simulink model "lqr_delay"  (R2017a)
settings: Solver=VariableStepAuto  StartTime=0.0  StopTime=4  RelTol=1e-3
values from neighbouring files (symbols this model uses):
  A_lq = [A7d B7d; 0 0 0 0]    [q13.m]
  B_lq = [0; 0; 0; 1]    [q13.m]
  C_lq = [C7d 0]    [q13.m]
  DCgain7 = D7d + C7cl*inv(eye(3)-A7cl)*B7d    [q13.m]    (also in q5.m; q5_reduced.m)
  DCgain_lq = D7d + C_lq_cl*inv(eye(4)-A_lq_cl)*B_lq    [q13.m]
  h7 = 0.08    [q13.m]    (also in q5.m = 0.006; q5_reduced.m)
undefined symbols (not defined in the file or in its folder): A7d, B7d, C7d, D5d, K7, K_lq
settings Model: Creator=Aleksandra  LastModifiedBy=Aleksandra

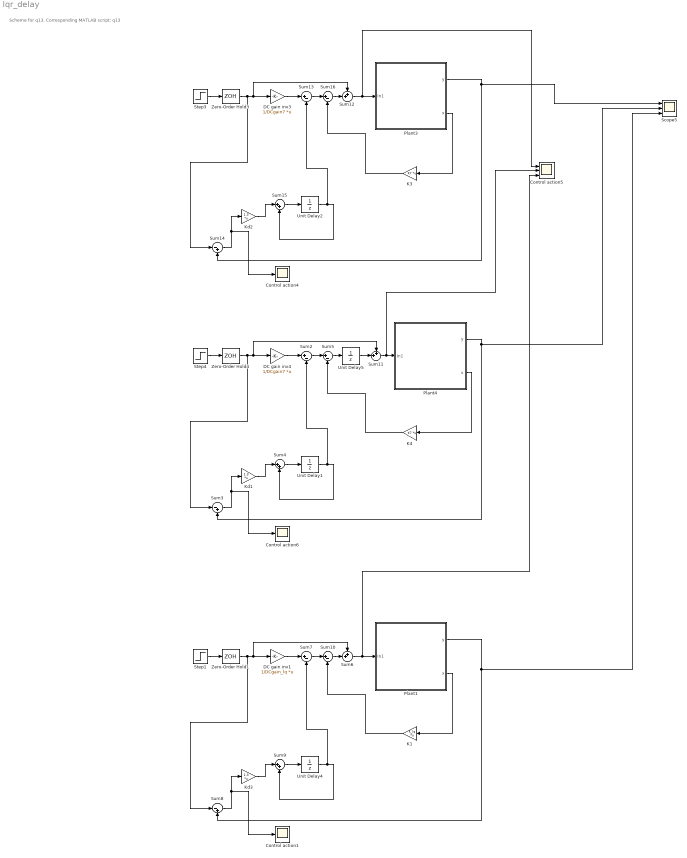
== system lqr_delay ==
  note: Scheme for q13.
      | Corresponding MATLAB script: q13
  Control action1 : Scope
  Control action4 : Scope
  Control action5 : Scope  NumInputPorts=3
  Control action6 : Scope
  DC gain inv1 : Gain  Gain=1/DCgain_lq  Multiplication=Matrix(K*u)
  DC gain inv3 : Gain  Gain=1/DCgain7  Multiplication=Matrix(K*u)
  DC gain inv4 : Gain  Gain=1/DCgain7  Multiplication=Matrix(K*u)
  K1 : Gain  Gain=K_lq  Multiplication=Matrix(K*u)
  K3 : Gain  Gain=K7  Multiplication=Matrix(K*u)
  K4 : Gain  Gain=K7  Multiplication=Matrix(K*u)
  Kd1 : Gain  Gain=1.3  Multiplication=Matrix(K*u)
  Kd2 : Gain  Gain=1.3  Multiplication=Matrix(K*u)
  Kd3 : Gain  Gain=1.3  Multiplication=Matrix(K*u)
  Plant1 : Subsystem
  Plant3 : Subsystem
  Plant4 : Subsystem
  Scope5 : Scope  NumInputPorts=3
  Step1 : Step  Time=0  SampleTime=0
  Step3 : Step  Time=0  SampleTime=0
  Step4 : Step  Time=0  SampleTime=0
  Sum{2,5,7,10,13,16} (6 alike) : Sum  Inputs=|+-
  Sum11 : Sum  Inputs=++|
  Sum12 : Sum  Inputs=++|
  Sum14 : Sum  Inputs=|-+
  Sum15 : Sum  Inputs=|++
  Sum3 : Sum  Inputs=|-+
  Sum4 : Sum  Inputs=|++
  Sum6 : Sum  Inputs=++|
  Sum8 : Sum  Inputs=|-+
  Sum9 : Sum  Inputs=|++
  Unit Delay{1..2,4..5} (4 alike) : UnitDelay  SampleTime=-1
  Zero-Order Hold1 : ZeroOrderHold  SampleTime=h7
  Zero-Order Hold3 : ZeroOrderHold  SampleTime=h7
  Zero-Order Hold4 : ZeroOrderHold  SampleTime=h7
  wires:
  Plant3/2(x) -> K3/1
  Sum13/1 -> Sum16/1
  Kd2/1 -> Sum15/1
  Step3/1 -> Zero-Order Hold3/1
  DC gain inv3/1 -> Sum13/1
  Sum14/1 -> Control action4/1, Kd2/1
  K3/1 -> Sum16/2
  Zero-Order Hold3/1 -> Sum14/1, Sum12/1, DC gain inv3/1
  Sum12/1 -> Control action5/1, Plant3/1(In1)
  Sum15/1 -> Unit Delay2/1
  Plant3/1(y) -> Scope5/1, Sum14/2
  Sum16/1 -> Sum12/2
  Unit Delay2/1 -> Sum13/2, Sum15/2
  Plant4/1(y) -> Scope5/2, Sum3/2
  Sum4/1 -> Unit Delay1/1
  Unit Delay5/1 -> Sum11/2
  Unit Delay1/1 -> Sum2/2, Sum4/2
  Zero-Order Hold4/1 -> Sum3/1, Sum11/1, DC gain inv4/1
  Sum5/1 -> Unit Delay5/1
  Sum3/1 -> Control action6/1, Kd1/1
  Step4/1 -> Zero-Order Hold4/1
  Plant4/2(x) -> K4/1
  DC gain inv4/1 -> Sum2/1
  Sum2/1 -> Sum5/1
  Kd1/1 -> Sum4/1
  K4/1 -> Sum5/2
  Sum11/1 -> Control action5/2, Plant4/1(In1)
  Plant1/1(y) -> Scope5/3, Sum8/2
  Sum9/1 -> Unit Delay4/1
  Sum6/1 -> Control action5/3, Plant1/1(In1)
  Unit Delay4/1 -> Sum7/2, Sum9/2
  Zero-Order Hold1/1 -> Sum8/1, Sum6/1, DC gain inv1/1
  Step1/1 -> Zero-Order Hold1/1
  Plant1/2(x) -> K1/1
  DC gain inv1/1 -> Sum7/1
  Sum7/1 -> Sum10/1
  Kd3/1 -> Sum9/1
  K1/1 -> Sum10/2
  Sum10/1 -> Sum6/2
  Sum8/1 -> Control action1/1, Kd3/1

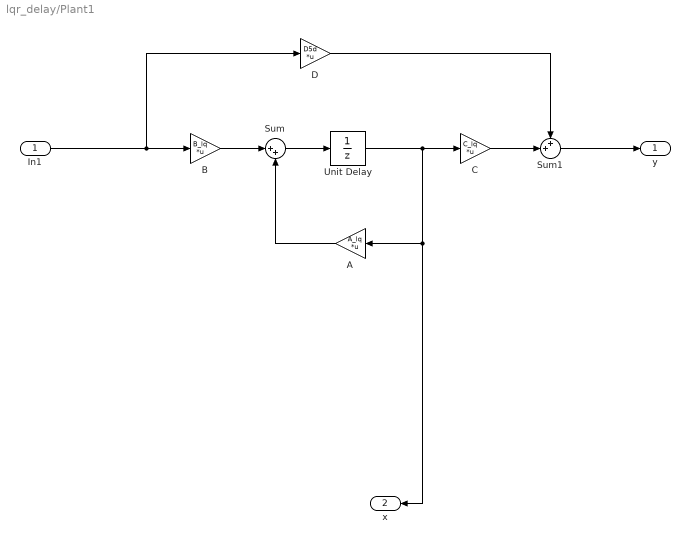
== system lqr_delay/Plant1 ==
  In1 : Inport
  A : Gain  Gain=A_lq  Multiplication=Matrix(K*u)
  B : Gain  Gain=B_lq  Multiplication=Matrix(K*u)
  C : Gain  Gain=C_lq  Multiplication=Matrix(K*u)
  D : Gain  Gain=D5d  Multiplication=Matrix(K*u)
  Sum : Sum  Inputs=|++
  Sum1 : Sum  Inputs=++|
  Unit Delay : UnitDelay  SampleTime=-1
  y : Outport
  x : Outport  Port=2
  wires:
  Sum/1 -> Unit Delay/1
  A/1 -> Sum/2
  D/1 -> Sum1/1
  C/1 -> Sum1/2
  Sum1/1 -> y/1
  B/1 -> Sum/1
  In1/1 -> D/1, B/1
  Unit Delay/1 -> x/1, A/1, C/1

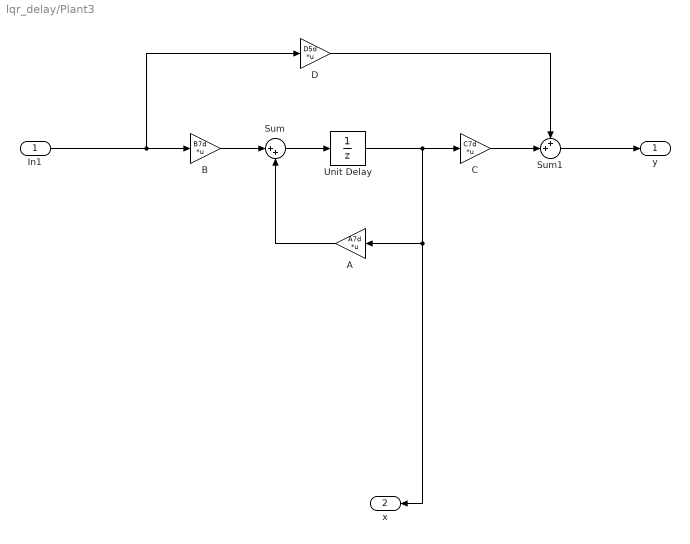
== system lqr_delay/Plant3 ==
  In1 : Inport
  A : Gain  Gain=A7d  Multiplication=Matrix(K*u)
  B : Gain  Gain=B7d  Multiplication=Matrix(K*u)
  C : Gain  Gain=C7d  Multiplication=Matrix(K*u)
  D : Gain  Gain=D5d  Multiplication=Matrix(K*u)
  Sum : Sum  Inputs=|++
  Sum1 : Sum  Inputs=++|
  Unit Delay : UnitDelay  SampleTime=-1
  y : Outport
  x : Outport  Port=2
  wires:
  Sum/1 -> Unit Delay/1
  A/1 -> Sum/2
  D/1 -> Sum1/1
  C/1 -> Sum1/2
  Sum1/1 -> y/1
  B/1 -> Sum/1
  In1/1 -> D/1, B/1
  Unit Delay/1 -> x/1, A/1, C/1

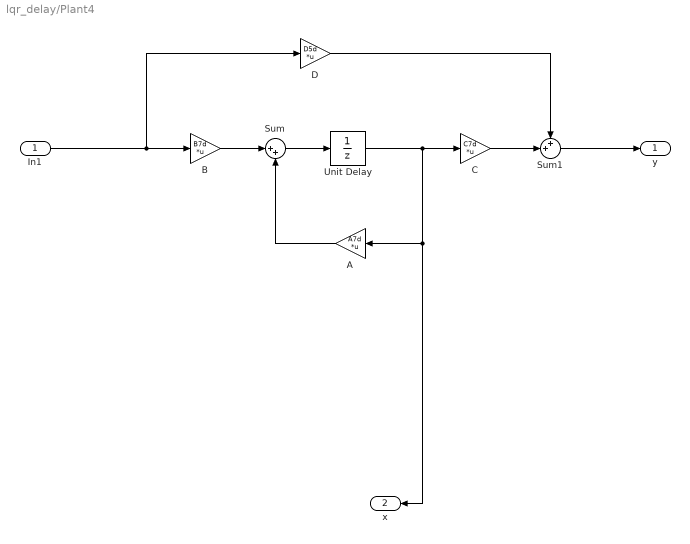
== system lqr_delay/Plant4 ==
  In1 : Inport
  A : Gain  Gain=A7d  Multiplication=Matrix(K*u)
  B : Gain  Gain=B7d  Multiplication=Matrix(K*u)
  C : Gain  Gain=C7d  Multiplication=Matrix(K*u)
  D : Gain  Gain=D5d  Multiplication=Matrix(K*u)
  Sum : Sum  Inputs=|++
  Sum1 : Sum  Inputs=++|
  Unit Delay : UnitDelay  SampleTime=-1
  y : Outport
  x : Outport  Port=2
  wires:
  Sum/1 -> Unit Delay/1
  A/1 -> Sum/2
  D/1 -> Sum1/1
  C/1 -> Sum1/2
  Sum1/1 -> y/1
  B/1 -> Sum/1
  In1/1 -> D/1, B/1
  Unit Delay/1 -> x/1, A/1, C/1
